simulink subsystem "Canard_Roll_Forcing_and_Damping"  (R2024b)
settings: Solver=VariableStepAuto  StartTime=0.0  StopTime=10.0  RelTol=1e-3
settings Model: Creator=trist  LastModifiedBy=trist

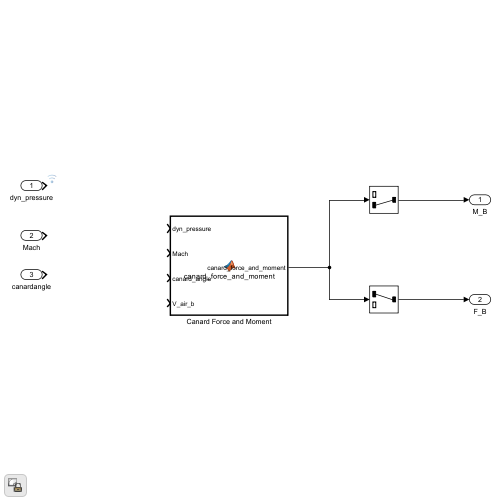
[thumbnail: Simulink's stored preview of the top-level diagram]
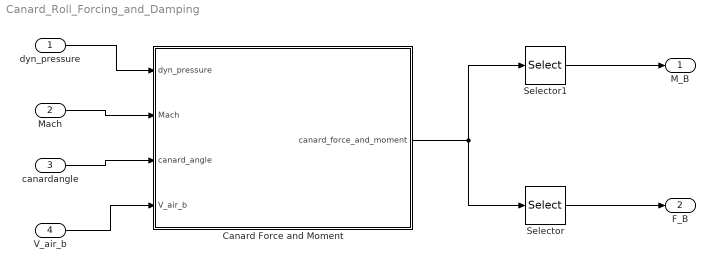
== system Canard_Roll_Forcing_and_Damping ==
  "dyn_pressure " : Inport
  "Mach " : Inport  Port=2
  canardangle : Inport  Port=3
  V_air_b : Inport  Port=4
  Canard Force and Moment : MATLAB Function  TreatAsAtomicUnit=on
  Selector : Selector  InputPortWidth=2  IndexOptions=Index vector (dialog)  Indices=[1]  OutputSizes=1
  Selector1 : Selector  InputPortWidth=2  IndexOptions=Index vector (dialog)  Indices=[2]  OutputSizes=1
  M_B : Outport  VectorParamsAs1DForOutWhenUnconnected=off
  F_B : Outport  Port=2  VectorParamsAs1DForOutWhenUnconnected=off
  wires:
  Canard Force and Moment/1(canard_force_and_moment) -> Selector1/1, Selector/1
  Selector1/1 -> M_B/1
  Selector/1 -> F_B/1
  V_air_b/1 -> Canard Force and Moment/4(V_air_b)
  canardangle/1 -> Canard Force and Moment/3(canard_angle)
  "Mach "/1 -> Canard Force and Moment/2(Mach)
  "dyn_pressure "/1 -> Canard Force and Moment/1(dyn_pressure)

== matlab function Canard_Roll_Forcing_and_Damping/Canard Force and Moment ==
  data: dyn_pressure input; Mach input; canard_angle input; V_air_b input; canard_force_and_moment output
function canard_force_and_moment = canard_dynamics(dyn_pressure, Mach, canard_angle, V_air_b)
    
    %supersonic correction:
    if Mach^2 > 0.75 && Mach^2 < 1.25
        ssc_factor = 2;
    else
        ssc_factor = 1/sqrt(abs(1-M^2));
    end

    canard_lever_arm = [0; 0; canard_dist_chord_mean]; %make all constants inputs
    V_rel_air = V_air_b - cross(omega_b, canard_lever_arm);
    theta_air = arccos(V_air_b/norm(V_rel_air));
    angle_of_attack = canard_angle - theta_air;
    lift_force = ssc_factor * dyn_pressure * canard_CLalpha * angle_of_attack * canard_area; %perhaps should be rocket area frontal? idk how our coeffs are defined
    drag_force = ssc_factor * dyn_pressure * canard_CDalpha * angle_of_attack * canard_area;
    force_air = [lift_force; drag_force]; 
    canard_force = [cos(-theta_air) -sin(-theta_air); sin(-theta_air) cos(-theta_air)] * force_air;
    canard_moment_x = canard_number * dot(canard_force, [1; 0]) * canard_dist_chord_mean;
    canard_force_x = canard_number * dot(canard_force, [0; 1]);
canard_force_and_moment = [canard_force_x, canard_moment_x];
